simulink model "fin_3ph_2lvl_autofilter"  (Simulink 7.5)
settings: Solver=ode45  StartTime=0.0  StopTime=0.5  RelTol=1e-3
libraries: powerlib x36, powerlib_extras x1
settings Model: Creator=IS  LastModifiedBy=IS
settings SolverCC: ZeroCrossAlgorithm=Adaptive

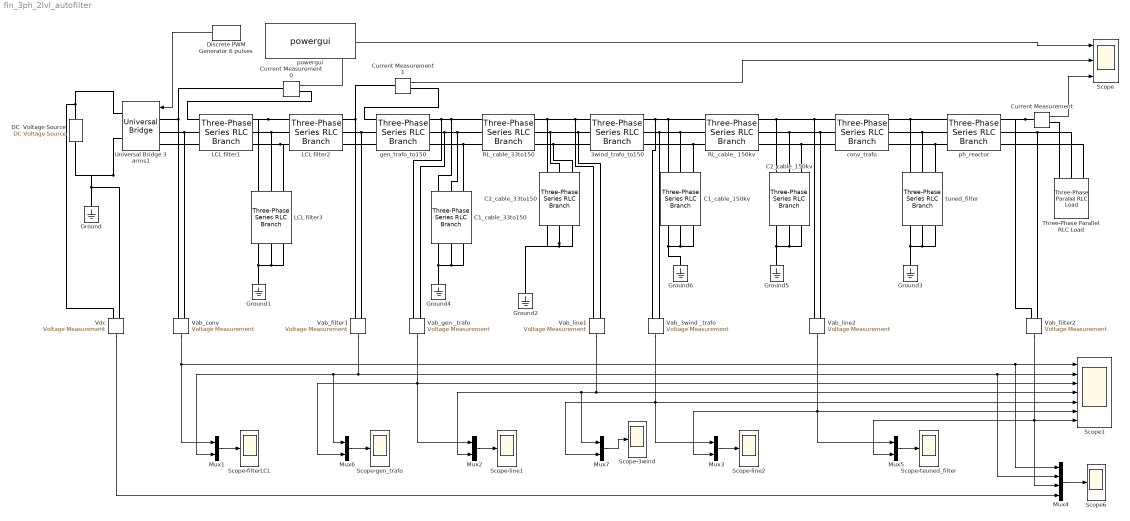
== system fin_3ph_2lvl_autofilter ==
  3wind_trafo_to150 : powerlib/Elements/Three-Phase Series RLC Branch  DialogController=POWERSYS.PowerSysDialog  PhysicalDomain=powersysdomain  SubClassName=unknown  LeftPortType=p1  RightPortType=p1  LConnTagsString=A|B|C  RConnTagsString=A|B|C  BranchType=L  Resistance=1  Inductance=2.27e-3  Capacitance=1e-6  Measurements=None
  C1_cable_150kv : powerlib/Elements/Three-Phase Series RLC Branch  DialogController=POWERSYS.PowerSysDialog  PhysicalDomain=powersysdomain  SubClassName=unknown  LeftPortType=p1  RightPortType=p1  LConnTagsString=A|B|C  RConnTagsString=A|B|C  BranchType=C  Resistance=1  Inductance=1e-3  Capacitance=5.2e-4  Measurements=None
  C1_cable_33to150 : powerlib/Elements/Three-Phase Series RLC Branch  DialogController=POWERSYS.PowerSysDialog  PhysicalDomain=powersysdomain  SubClassName=unknown  LeftPortType=p1  RightPortType=p1  LConnTagsString=A|B|C  RConnTagsString=A|B|C  BranchType=C  Resistance=1  Inductance=1e-3  Capacitance=9.71e-7  Measurements=None
  C2_cable_150kv : powerlib/Elements/Three-Phase Series RLC Branch  DialogController=POWERSYS.PowerSysDialog  PhysicalDomain=powersysdomain  SubClassName=unknown  LeftPortType=p1  RightPortType=p1  LConnTagsString=A|B|C  RConnTagsString=A|B|C  BranchType=C  Resistance=1  Inductance=1e-3  Capacitance=5.2e-4  Measurements=None
  C2_cable_33to150 : powerlib/Elements/Three-Phase Series RLC Branch  DialogController=POWERSYS.PowerSysDialog  PhysicalDomain=powersysdomain  SubClassName=unknown  LeftPortType=p1  RightPortType=p1  LConnTagsString=A|B|C  RConnTagsString=A|B|C  BranchType=C  Resistance=1  Inductance=1e-3  Capacitance=9.71e-7  Measurements=None
  Current Measurement : powerlib/Measurements/Current Measurement  DialogController=POWERSYS.PowerSysDialog  SystemSampleTime=-1  PhasorSimulation=off  OutputType=Complex  PSBequivalent=0
  Current Measurement0 : powerlib/Measurements/Current Measurement  DialogController=POWERSYS.PowerSysDialog  SystemSampleTime=-1  PhasorSimulation=off  OutputType=Complex  PSBequivalent=0
  Current Measurement1 : powerlib/Measurements/Current Measurement  DialogController=POWERSYS.PowerSysDialog  SystemSampleTime=-1  PhasorSimulation=off  OutputType=Complex  PSBequivalent=0
  DC  Voltage Source : powerlib/Electrical Sources/DC Voltage Source  DialogController=POWERSYS.PowerSysDialog  SystemSampleTime=-1  Amplitude=212e3  Measurements=None
  Discrete PWM Generator 6 pulses : powerlib_extras/Discrete  Control Blocks/Discrete PWM Generator  DialogController=POWERSYS.PowerSysDialog  SystemSampleTime=-1  GeneratorMode="3-arm  bridge (6 pulses)"  Fc=1000  Ts=0.000001  Internal=on  mIndex=1  Freq=50  Phase=0
  Ground{,1..6} (7 alike) : powerlib/Elements/Ground  DialogController=POWERSYS.PowerSysDialog  PhysicalDomain=powersysdomain  SubClassName=unknown  LeftPortType=p1  RightPortType=p1  LConnTagsString=a
  LCL filter1 : powerlib/Elements/Three-Phase Series RLC Branch  DialogController=POWERSYS.PowerSysDialog  PhysicalDomain=powersysdomain  SubClassName=unknown  LeftPortType=p1  RightPortType=p1  LConnTagsString=A|B|C  RConnTagsString=A|B|C  BranchType=RL  Resistance=0.2  Inductance=3.41e-3  Capacitance=1e-6  Measurements=None
  LCL filter2 : powerlib/Elements/Three-Phase Series RLC Branch  DialogController=POWERSYS.PowerSysDialog  PhysicalDomain=powersysdomain  SubClassName=unknown  LeftPortType=p1  RightPortType=p1  LConnTagsString=A|B|C  RConnTagsString=A|B|C  BranchType=RL  Resistance=0.2  Inductance=1.82e-3  Capacitance=1e-6  Measurements=None
  LCL filter3 : powerlib/Elements/Three-Phase Series RLC Branch  DialogController=POWERSYS.PowerSysDialog  PhysicalDomain=powersysdomain  SubClassName=unknown  LeftPortType=p1  RightPortType=p1  LConnTagsString=A|B|C  RConnTagsString=A|B|C  BranchType=RC  Resistance=5  Inductance=1e-3  Capacitance=5.24e-5  Measurements=None
  Mux{1..3,5..7} (6 alike) : Mux  Inputs=2
  Mux4 : Mux
  RL_cable_ 150kv : powerlib/Elements/Three-Phase Series RLC Branch  DialogController=POWERSYS.PowerSysDialog  PhysicalDomain=powersysdomain  SubClassName=unknown  LeftPortType=p1  RightPortType=p1  LConnTagsString=A|B|C  RConnTagsString=A|B|C  BranchType=RL  Resistance=5.6e-2  Inductance=1e-3  Capacitance=1e-6  Measurements=None
  RL_cable_33to150 : powerlib/Elements/Three-Phase Series RLC Branch  DialogController=POWERSYS.PowerSysDialog  PhysicalDomain=powersysdomain  SubClassName=unknown  LeftPortType=p1  RightPortType=p1  LConnTagsString=A|B|C  RConnTagsString=A|B|C  BranchType=RL  Resistance=2.19e-2  Inductance=1.07e-3  Capacitance=1e-6  Measurements=None
  Scope : Scope  NumInputPorts=3
      settings: YMin=-175000~24.75~-5  YMax=200000~28.25~5  SaveName=two_lvl_currents
  Scope-3wind : Scope
      settings: TimeRange=0.5  YMin=-500  YMax=500  SaveName=psb3phPWM1_str7  MaxDataPoints=50000
  Scope-filterLCL : Scope
      settings: TimeRange=0.3  YMin=-225000  YMax=225000  SaveName=psb3phPWM1_str1  MaxDataPoints=50000
  Scope-gen_trafo : Scope
      settings: TimeRange=0.5  YMin=-500  YMax=500  SaveName=psb3phPWM1_str6  MaxDataPoints=50000
  Scope-line1 : Scope
      settings: TimeRange=0.5  YMin=-500  YMax=500  SaveName=psb3phPWM1_str2  MaxDataPoints=50000
  Scope-line2 : Scope
      settings: TimeRange=0.5  YMin=-500  YMax=500  SaveName=psb3phPWM1_str3  MaxDataPoints=50000
  Scope-teuned_filter : Scope
      settings: TimeRange=0.5  YMin=-500  YMax=500  SaveName=psb3phPWM1_str4  MaxDataPoints=50000
  Scope1 : Scope  NumInputPorts=7
      settings: TimeRange=0.5  YMin=-500~-400~-5~-5~-5~-5~-5  YMax=500~500~5~5~5~5~5  SaveName=two_lvl_volgates  MaxDataPoints=30000
  Scope6 : Scope
      settings: TimeRange=0.5  YMin=-500  YMax=500  SaveName=psb3phPWM1_str5  MaxDataPoints=20000
  Three-Phase Parallel RLC Load : powerlib/Elements/Three-Phase Parallel RLC Load  DialogController=POWERSYS.PowerSysDialog  PhysicalDomain=powersysdomain  SubClassName=unknown  LeftPortType=p1  RightPortType=p1  LConnTagsString=A|B|C  Configuration=Delta  NominalVoltage=150e3  NominalFrequency=50  ActivePower=1000e3  InductivePower=100000  CapacitivePower=100000  Measurements=None
  Universal Bridge 3 arms1 : powerlib/Power Electronics/Universal Bridge  DialogController=POWERSYS.PowerSysDialog  SystemSampleTime=-1  Arms=3  SnubberResistance=10000  SnubberCapacitance=inf  Device=IGBT / Diodes  Ron=1e-4  Lon=0  ForwardVoltages="[  1  1  ]"  ForwardVoltage=.8  GTOparameters=[ 10e-6 , 20e-6 ]  IGBTparameters=[ 1e-6 , 2e-6 ]  Measurements=None  Measurements_2=None  converterType=Rectifier
  Vab_3wind _trafo : powerlib/Measurements/Voltage Measurement  Tag=PoWeRsYsTeMmEaSuReMeNt  DialogController=POWERSYS.PowerSysDialog  SystemSampleTime=-1  PhasorSimulation=off  OutputType=Magnitude  PSBequivalent=0
  Vab_conv : powerlib/Measurements/Voltage Measurement  Tag=PoWeRsYsTeMmEaSuReMeNt  DialogController=POWERSYS.PowerSysDialog  SystemSampleTime=-1  PhasorSimulation=off  OutputType=Magnitude  PSBequivalent=0
  Vab_filter1 : powerlib/Measurements/Voltage Measurement  Tag=PoWeRsYsTeMmEaSuReMeNt  DialogController=POWERSYS.PowerSysDialog  SystemSampleTime=-1  PhasorSimulation=off  OutputType=Magnitude  PSBequivalent=0
  Vab_filter2 : powerlib/Measurements/Voltage Measurement  Tag=PoWeRsYsTeMmEaSuReMeNt  DialogController=POWERSYS.PowerSysDialog  SystemSampleTime=-1  PhasorSimulation=off  OutputType=Magnitude  PSBequivalent=0
  Vab_gen _trafo : powerlib/Measurements/Voltage Measurement  Tag=PoWeRsYsTeMmEaSuReMeNt  DialogController=POWERSYS.PowerSysDialog  SystemSampleTime=-1  PhasorSimulation=off  OutputType=Magnitude  PSBequivalent=0
  Vab_line1 : powerlib/Measurements/Voltage Measurement  Tag=PoWeRsYsTeMmEaSuReMeNt  DialogController=POWERSYS.PowerSysDialog  SystemSampleTime=-1  PhasorSimulation=off  OutputType=Magnitude  PSBequivalent=0
  Vab_line2 : powerlib/Measurements/Voltage Measurement  Tag=PoWeRsYsTeMmEaSuReMeNt  DialogController=POWERSYS.PowerSysDialog  SystemSampleTime=-1  PhasorSimulation=off  OutputType=Magnitude  PSBequivalent=0
  Vdc : powerlib/Measurements/Voltage Measurement  Tag=PoWeRsYsTeMmEaSuReMeNt  DialogController=POWERSYS.PowerSysDialog  SystemSampleTime=-1  PhasorSimulation=off  OutputType=Magnitude  PSBequivalent=0
  conv_trafo : powerlib/Elements/Three-Phase Series RLC Branch  DialogController=POWERSYS.PowerSysDialog  PhysicalDomain=powersysdomain  SubClassName=unknown  LeftPortType=p1  RightPortType=p1  LConnTagsString=A|B|C  RConnTagsString=A|B|C  BranchType=L  Resistance=1  Inductance=1.93e-2  Capacitance=1e-6  Measurements=None
  gen_trafo_to150 : powerlib/Elements/Three-Phase Series RLC Branch  DialogController=POWERSYS.PowerSysDialog  PhysicalDomain=powersysdomain  SubClassName=unknown  LeftPortType=p1  RightPortType=p1  LConnTagsString=A|B|C  RConnTagsString=A|B|C  BranchType=L  Resistance=1  Inductance=1.47e-4  Capacitance=1e-6  Measurements=None
  ph_reactor : powerlib/Elements/Three-Phase Series RLC Branch  DialogController=POWERSYS.PowerSysDialog  PhysicalDomain=powersysdomain  SubClassName=unknown  LeftPortType=p1  RightPortType=p1  LConnTagsString=A|B|C  RConnTagsString=A|B|C  BranchType=L  Resistance=1  Inductance=1.93e-2  Capacitance=1e-6  Measurements=None
  powergui : powerlib/powergui  Priority=1  SystemSampleTime=-1  SimulationMode=Discrete  SampleTime=5e-6  frequency=60  SPID=off  DisableSnubberDevices=off  DisableRonSwitches=off  DisableVfSwitches=off  SwTol=0  Interpol=off  frequencyindice=0  echomessages=off  HookPort=off  DisplayEquations=off  FunctionMessages=off  EnableUseOfTLC=off  x0status=blocks  RestoreLinks=warning  ResistiveCurrentMeasurement=off  Ylog=off  Xlog=on  ShowGrid=off  save=off  variable=ZData  structure=two_lvl_volgates  ZoomFFT=off  StartTime=0.36  cycles=7  DisplayStyle=1  fundamental=50  FreqAxis=on  MaxFrequency=5000  frequencyindicesteady=1  display=off  methode=off
  tuned_filter : powerlib/Elements/Three-Phase Series RLC Branch  DialogController=POWERSYS.PowerSysDialog  PhysicalDomain=powersysdomain  SubClassName=unknown  LeftPortType=p1  RightPortType=p1  LConnTagsString=A|B|C  RConnTagsString=A|B|C  BranchType=C  Resistance=1  Inductance=1e-3  Capacitance=5.66e-6  Measurements=None
  wires:
  Discrete PWM Generator 6 pulses/1 -> Universal Bridge 3 arms1/1
  Vab_conv/1 -> Scope1/1, Mux4/1, Mux1/1
  Vab_filter1/1 -> Mux1/2, Mux6/1, Scope1/2, Mux4/2
  Vab_gen _trafo/1 -> Scope1/3, Mux2/1, Mux6/2
  Vab_line1/1 -> Scope1/4, Mux2/2, Mux7/1
  Vab_3wind _trafo/1 -> Scope1/5, Mux3/1, Mux7/2
  Vab_line2/1 -> Scope1/6, Mux3/2, Mux5/1
  Vab_filter2/1 -> Scope1/7, Mux5/2, Mux4/3
  Mux4/1 -> Scope6/1
  Mux1/1 -> Scope-filterLCL/1
  Mux2/1 -> Scope-line1/1
  Mux3/1 -> Scope-line2/1
  Mux5/1 -> Scope-teuned_filter/1
  Vdc/1 -> Mux4/4
  Mux6/1 -> Scope-gen_trafo/1
  Mux7/1 -> Scope-3wind/1
  Current Measurement/1 -> Scope/3
  Current Measurement1/1 -> Scope/2
  Current Measurement0/1 -> Scope/1
  connections:
  DC  Voltage Source/RConn1 -- Universal Bridge 3 arms1/RConn1 -- Vdc/LConn1
  Ground/LConn1 -- Vdc/LConn2 -- Universal Bridge 3 arms1/RConn2 -- DC  Voltage Source/LConn1
  gen_trafo_to150/LConn2 -- LCL filter2/RConn2 -- Vab_filter1/LConn2
  tuned_filter/RConn1 -- Ground3/LConn1 -- tuned_filter/RConn2 -- tuned_filter/RConn3
  ph_reactor/LConn3 -- conv_trafo/RConn3 -- tuned_filter/LConn3
  ph_reactor/LConn2 -- conv_trafo/RConn2 -- tuned_filter/LConn2
  conv_trafo/RConn1 -- ph_reactor/LConn1 -- tuned_filter/LConn1
  Vab_filter2/LConn1 -- ph_reactor/RConn1 -- Current Measurement/LConn1
  Three-Phase Parallel RLC Load/LConn2 -- ph_reactor/RConn2 -- Vab_filter2/LConn2
  ph_reactor/RConn3 -- Three-Phase Parallel RLC Load/LConn3
  LCL filter1/RConn1 -- LCL filter3/LConn1 -- LCL filter2/LConn1
  LCL filter2/LConn2 -- LCL filter3/LConn2 -- LCL filter1/RConn2
  LCL filter2/LConn3 -- LCL filter3/LConn3 -- LCL filter1/RConn3
  LCL filter3/RConn3 -- LCL filter3/RConn2 -- LCL filter3/RConn1 -- Ground1/LConn1
  LCL filter2/RConn3 -- gen_trafo_to150/LConn3
  LCL filter2/RConn1 -- Vab_filter1/LConn1 -- Current Measurement1/LConn1
  Universal Bridge 3 arms1/LConn1 -- Vab_conv/LConn1 -- Current Measurement0/LConn1
  LCL filter1/LConn2 -- Universal Bridge 3 arms1/LConn2 -- Vab_conv/LConn2
  LCL filter1/LConn3 -- Universal Bridge 3 arms1/LConn3
  C2_cable_33to150/LConn1 -- RL_cable_33to150/RConn1 -- 3wind_trafo_to150/LConn1 -- Vab_line1/LConn1
  RL_cable_33to150/RConn2 -- C2_cable_33to150/LConn2 -- 3wind_trafo_to150/LConn2 -- Vab_line1/LConn2
  gen_trafo_to150/RConn2 -- RL_cable_33to150/LConn2 -- C1_cable_33to150/LConn2 -- Vab_gen _trafo/LConn2
  RL_cable_33to150/LConn3 -- C1_cable_33to150/LConn3 -- gen_trafo_to150/RConn3
  3wind_trafo_to150/LConn3 -- RL_cable_33to150/RConn3 -- C2_cable_33to150/LConn3
  RL_cable_33to150/LConn1 -- gen_trafo_to150/RConn1 -- Vab_gen _trafo/LConn1 -- C1_cable_33to150/LConn1
  C2_cable_150kv/RConn3 -- C2_cable_150kv/RConn2 -- Ground5/LConn1 -- C2_cable_150kv/RConn1
  Ground6/LConn1 -- C1_cable_150kv/RConn3 -- C1_cable_150kv/RConn2 -- C1_cable_150kv/RConn1
  C2_cable_150kv/LConn1 -- RL_cable_ 150kv/RConn1 -- conv_trafo/LConn1 -- Vab_line2/LConn1
  C2_cable_150kv/LConn2 -- RL_cable_ 150kv/RConn2 -- conv_trafo/LConn2 -- Vab_line2/LConn2
  3wind_trafo_to150/RConn2 -- RL_cable_ 150kv/LConn2 -- C1_cable_150kv/LConn2 -- Vab_3wind _trafo/LConn2
  3wind_trafo_to150/RConn3 -- RL_cable_ 150kv/LConn3 -- C1_cable_150kv/LConn3
  conv_trafo/LConn3 -- RL_cable_ 150kv/RConn3 -- C2_cable_150kv/LConn3
  3wind_trafo_to150/RConn1 -- RL_cable_ 150kv/LConn1 -- C1_cable_150kv/LConn1 -- Vab_3wind _trafo/LConn1
  C1_cable_33to150/RConn2 -- C1_cable_33to150/RConn1 -- Ground4/LConn1 -- C1_cable_33to150/RConn3
  Current Measurement/RConn1 -- Three-Phase Parallel RLC Load/LConn1
  Current Measurement1/RConn1 -- gen_trafo_to150/LConn1
  C2_cable_33to150/RConn2 -- C2_cable_33to150/RConn3 -- C2_cable_33to150/RConn1 -- Ground2/LConn1
  LCL filter1/LConn1 -- Current Measurement0/RConn1
